simulink model "m000_UseCommon"  (R2022a)
settings: Solver=VariableStepAuto  StartTime=0.0  StopTime=10.0  RelTol=1e-3
settings Model: Creator=Admin  LastModifiedBy=Admin

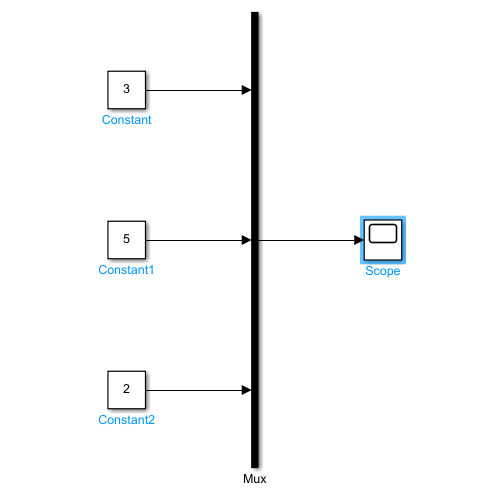
[thumbnail: Simulink's stored preview of the top-level diagram]
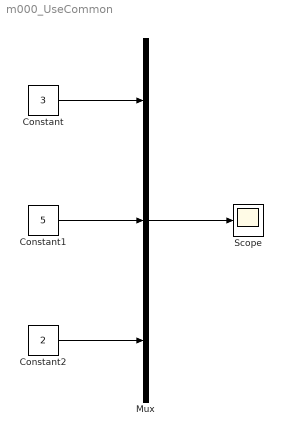
== system m000_UseCommon ==
  Constant : Constant  Value=3
  Constant1 : Constant  Value=5
  Constant2 : Constant  Value=2
  Mux : Mux  Inputs=3
  Scope : Scope
  wires:
  Constant/1 -> Mux/1
  Constant2/1 -> Mux/3
  Mux/1 -> Scope/1
  Constant1/1 -> Mux/2
